simulink model "ForIterator2"  (R2017b)
settings: Solver=FixedStepDiscrete  StartTime=0.0  StopTime=10.0  FixedStep=0.200000  RelTol=1e-3  EnableMultiTasking=on
settings Model: Creator=ktrinh  LastModifiedBy=hbourbou
settings DataIOCC: SaveFormat=Structure
settings OptimizationCC: LifeSpan=inf
settings DebuggingCC: SFUnexpectedBacktrackingDiag=warning  SFNoUnconditionalDefaultTransitionDiag=warning  SFExecutionAtInitializationDiag=none
settings HardwareCC: ProdBitPerSizeT=32  ProdBitPerPtrDiffT=32  ProdWordSize=32  ProdHWDeviceType=Specified
settings CodeAppCC: StateflowObjectComments=on
settings GRTTargetCC: TargetLangStandard=C89/C90 (ANSI)  GeneratePreprocessorConditionals=Disable all
settings ConfigComp: CovMetricSettings=dw  CovHtmlReporting=on  CovSaveCumulativeToWorkspaceVar=on  CovSaveSingleToWorkspaceVar=on  CovExternalEMLEnable=off

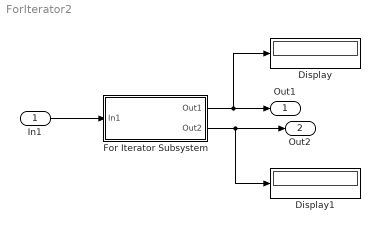
== system ForIterator2 ==
  In1 : Inport
  Display : Display
  Display1 : Display
  For Iterator Subsystem : Subsystem  TreatAsAtomicUnit=on
  Out1 : Outport
  Out2 : Outport  Port=2
  wires:
  In1/1 -> For Iterator Subsystem/1(In1)
  For Iterator Subsystem/1(Out1) -> Display/1, Out1/1
  For Iterator Subsystem/2(Out2) -> Display1/1, Out2/1

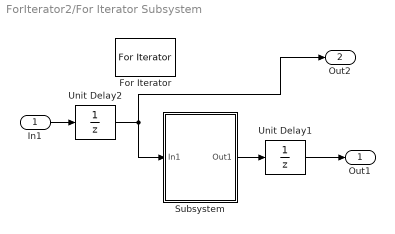
== system ForIterator2/For Iterator Subsystem ==
  In1 : Inport  OutDataTypeStr=double  PortDimensions=1
  For Iterator : ForIterator  IterationLimit=3  ShowIterationPort=off
  Subsystem : Subsystem
  Unit Delay1 : UnitDelay  SampleTime=-1
  Unit Delay2 : UnitDelay  SampleTime=-1
  Out1 : Outport
  Out2 : Outport  Port=2
  wires:
  In1/1 -> Unit Delay2/1
  Unit Delay1/1 -> Out1/1
  Unit Delay2/1 -> Subsystem/1(In1), Out2/1
  Subsystem/1(Out1) -> Unit Delay1/1

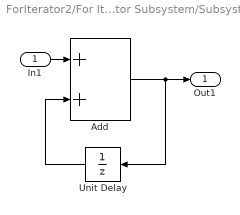
== system ForIterator2/For Iterator Subsystem/Subsystem ==
  In1 : Inport
  Add : Sum
  Unit Delay : UnitDelay  SampleTime=-1
  Out1 : Outport
  wires:
  In1/1 -> Add/1
  Unit Delay/1 -> Add/2
  Add/1 -> Out1/1, Unit Delay/1
